simulink model "Arrays1_PP"  (Simulink 9.0)
settings: Solver=FixedStepDiscrete  StartTime=0.0  StopTime=19800  FixedStep=200  RelTol=1e-3  EnableMultiTasking=on
model workspace (MAT data in the model file):
  already_pp : num (value not decoded)
settings Model: SuppressorTable=22 serialization::archive 11 0 6 0 0 0 0 0  Creator=scaife  LastModifiedBy=hbourbou  ExtModeAutoUpdateStatusClock=off
settings DataIOCC: ExternalInput=input_dataset  LimitDataPoints=on  SaveFormat=Dataset  SignalLoggingSaveFormat=ModelDataLogs  SaveState=on  SignalLoggingName=sigsOut
settings DebuggingCC: AlgebraicLoopMsg=error  SaveWithParameterizedLinksMsg=none  SignalResolutionControl=TryResolveAllWithWarning  MultiTaskDSMMsg=warning  MultiTaskCondExecSysMsg=none  StrictBusMsg=None
settings HardwareCC: TargetUnknown=on
settings SFSimCC: SimParseCustomCode=off
settings GRTTargetCC: GeneratePreprocessorConditionals=Disable all  CombineOutputUpdateFcns=off  GRTInterface=on  ExtMode=on

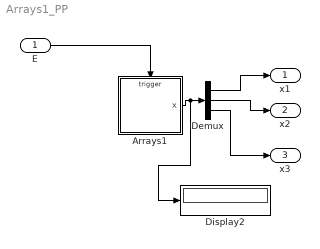
== system Arrays1_PP ==
  E : Inport
  Arrays1 : Stateflow chart  TreatAsAtomicUnit=on
  Demux : Demux  Outputs=3
  Display2 : Display
  x1 : Outport
  x2 : Outport  Port=2
  x3 : Outport  Port=3
  wires:
  E/1 -> Arrays1/Trigger
  Arrays1/1(x) -> Display2/1, Demux/1
  Demux/1 -> x1/1
  Demux/2 -> x2/1
  Demux/3 -> x3/1

== stateflow chart Arrays1 ==
  state A/
    en:
    i = 3;
    x = x([3, 1, 2]) + 1;
  state B/
    en:x(2) = x(2) + 1;
  state C/
    en:x(3) = x(3) + 1;
  (default) -> A
  A -> B : E
  C -> A : E
  B -> C : E
  data: x output int32 size=3 [0..100] =int32([1 ;2 ;3]); i local double
  events: E input RISING_EDGE_EVENT
